simulink model "uwb_6_delay_mult_optim"  (R2025a)
settings: Solver=VariableStepAuto  StartTime=0.0  StopTime=1.6e-6  RelTol=1e-3
undefined symbols (not defined in the file or in its folder): j
libraries: commrfcorlib x1, commchan3 x1, commdigbbndpm3 x1, dspstat3 x1
settings Model: Creator=IWMAI  LastModifiedBy=IWMAI

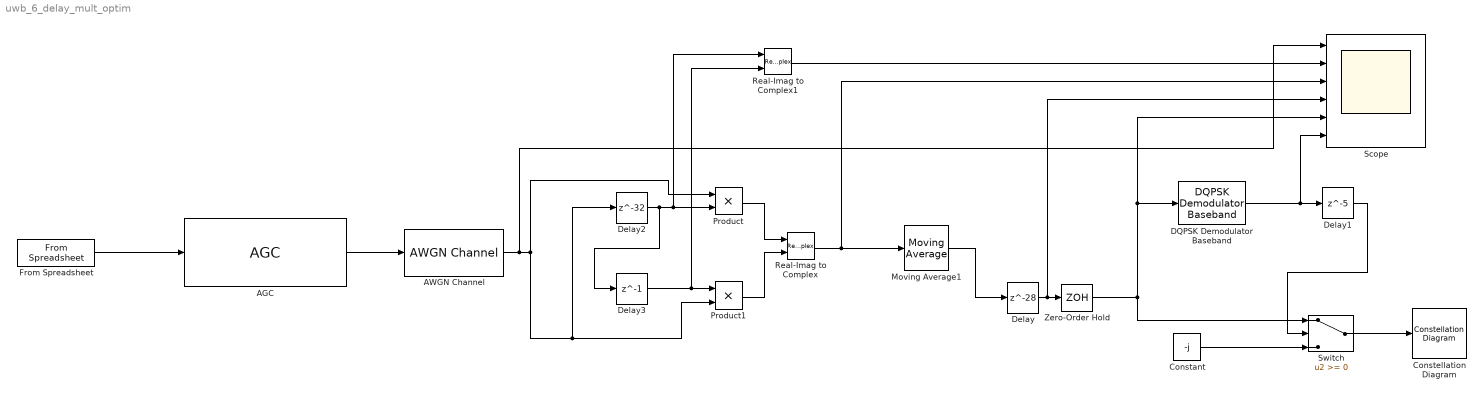
== system uwb_6_delay_mult_optim ==
  AGC : commrfcorlib/AGC  LegacyMode=off  DetectorMethod=Rectifier  LoopMethod=Linear  UpdatePeriod=100  StepSize=0.1  AdaptationStepSize=0.01  DesiredOutputPower=1/2  AveragingLength=64  MaximumGain=30  MaxPowerGain=60  GainOutputPort=off  InputPowerOutputPort=off  SimulateUsing=Interpreted execution
  AWGN Channel : commchan3/AWGN Channel  LegacyMode=off  NoiseMethod="Signal to noise ratio  (SNR)"  noiseMode="Signal to noise ratio  (SNR)"  EbNo=10  EsNo=10  SNR=15  BitsPerSymbol=1  SignalPower=1  SpecifySymbolPeriod=off  SamplesPerSymbol=1  SymbolPeriod=1  VarianceSource=Parameter  Variance=1  RandomStream=Global stream  Seed=67  SimulateUsing=Code generation
  Constant : Constant  Value=-j
  Constellation Diagram : ConstellationDiagram  WindowPosition=[609.000000,-743.000000,487.000000,337.000000,]  ScopeFrameLocation=window  SymbolsToDisplaySource=Property  SymbolsToDisplay=2500  ReferenceConstellation=QPSK  XLimits=[-2.067197093509777,2.1540515483355467]  YLimits=[-2.067197093509777,2.1540515483355467]  AxesLimits=[-2.067197093509777,2.1540515483355467]  EnableMeasurements=on  DefaultConfigurationName=comm.scopes.ConstellationDiagramBlockCfg
  DQPSK Demodulator Baseband : commdigbbndpm3/DQPSK Demodulator Baseband  OutType=Integer  Dec=Gray  Ph=0  outDtype1=Inherit via internal rule  outDtype2=Inherit via internal rule
  Delay : Delay  DelayLength=28
  Delay1 : Delay  DelayLength=5  InitialCondition=-1
  Delay2 : Delay  DelayLength=32
  Delay3 : Delay  DelayLength=1
  From Spreadsheet : FromSpreadsheet  FileName=C:\Users\IWMAI\University of Toronto\Yu Huang - Summer-2025-sharted\Yongkang\v3_250617\csv\data_zero_time.csv  SheetName=data_zero_time  SampleTime=1/16e9  ExtrapolationBeforeFirstDataPoint=Hold first value  InterpolationWithinTimeRange=Zero order hold  ExtrapolationAfterLastDataPoint=Hold last value
  Moving Average1 : dspstat3/Moving Average  Method=Sliding window  ForgettingFactorPort=off  SpecifyWindowLength=on  WindowLength=8  OverlapLength=7  AllowArbitraryInputLength=off  ForgettingFactor=0.9  SimulateUsing=Interpreted execution
  Product : Product
  Product1 : Product
  Real-Imag to Complex : RealImagToComplex
  Real-Imag to Complex1 : RealImagToComplex
  Scope : Scope  NumInputPorts=6
      settings: ActiveDisplayYMinimum=-2.8853361781018032  ActiveDisplayYMaximum=2.6693087362148233
  Switch : Switch  SaturateOnIntegerOverflow=off  InputSameDT=off
  Zero-Order Hold : ZeroOrderHold  SampleTime=1/500e6
  wires:
  Delay2/1 -> Delay3/1, Real-Imag to Complex1/1, Product/2
  Delay3/1 -> Real-Imag to Complex1/2, Product1/1
  Product/1 -> Real-Imag to Complex/1
  Product1/1 -> Real-Imag to Complex/2
  Real-Imag to Complex/1 -> Scope/3, Moving Average1/1
  Moving Average1/1 -> Delay/1
  Zero-Order Hold/1 -> Switch/1, DQPSK Demodulator Baseband/1, Scope/5
  Delay/1 -> Scope/4, Zero-Order Hold/1
  DQPSK Demodulator Baseband/1 -> Delay1/1, Scope/6
  Real-Imag to Complex1/1 -> Scope/2
  From Spreadsheet/1 -> AGC/1
  AWGN Channel/1 -> Scope/1, Product/1, Delay2/1, Product1/2
  AGC/1 -> AWGN Channel/1
  Delay1/1 -> Switch/2
  Switch/1 -> Constellation Diagram/1
  Constant/1 -> Switch/3
